simulink model "SF5_3_4_jc0733"  (R2016b)
settings: Solver=VariableStepAuto  StartTime=0.0  StopTime=10.0  RelTol=1e-3
settings Model: Creator=amyyang  LastModifiedBy=amyyang

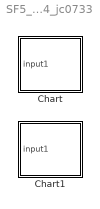
== system SF5_3_4_jc0733 ==
  Chart : Stateflow chart  TreatAsAtomicUnit=on
  Chart1 : Stateflow chart  TreatAsAtomicUnit=on

== stateflow chart SF5_3_4_jc0733/Chart1 ==
  state AA
    ex:
    param3 = 50;
    en,du:
    param1 = param1+param2;
    en:
    param1 = 0;
    param2 = 1;
    param3 = 10;
  note: en被放到了ex后面；
      |
      | 组合命令，放在最上面或者最下面；
  state AB
    en:
    param1 = 10;
    param2 = 2;
    en,du:
    param1 = param1+param2;
  (default) -> AA : {
      |  param3 = 0;
      | }
  AA -> AB : [(input1+param1)>param3]
  AB -> AA : [(input1+param1)>param3]
  data: input1 input; param1 local double; param2 local double; param3 local double

== stateflow chart SF5_3_4_jc0733/Chart ==
  state AA
    en:
    param1 = 0;
    param2 = 0;
    param3 = 0;
    du:
    param1 = param1+param2;
  state AB
    en:
    param1 = 10;
    param2 = 2;
    en,du:
    param1 = param1+param2;
  (default) -> AA
  AA -> AB : [(input1+param1)>param3]
  AB -> AA : [(input1+param1)>param3]
  data: input1 input; param1 local double; param2 local double; param3 local double
